simulink library "cyclopsLib"  (R2020a)
settings: Solver=VariableStepAuto  StartTime=0.0  StopTime=10.0  RelTol=1e-3
values from neighbouring files (symbols this model uses):
  agc_delay_lag = 32    [rev0BB_setup.m]
  agc_detector_coef = ones(1,agc_detector_taps)./agc_detector_taps    [rev0BB_setup.m]
  agc_sat_low = -agcSaturation    (= -12)    [rev0BB_setup.m]
  agc_sat_up = agcSaturation    (= 12)    [rev0BB_setup.m]
  agcDesired = 0    [rev0BB_setup.m]
  agcExpDomain = agcSaturation    (= 12)    [rev0BB_setup.m]
  agcExpResolution = 2^-3    (= 0.125)    [rev0BB_setup.m]
  agcPwrAvgNum = 128    [rev0BB_setup.m]
  agcSettleThresh = 0.65    [rev0BB_setup.m]
  agcStep = 2^-8    (= 0.00390625)    [rev0BB_setup.m]
  atanDomain = 5    [rev0BB_setup.m]
  atanResolution = 2^-9    (= 0.001953125)    [rev0BB_setup.m]
  bitsPerSymbolHeader = log2(radixHeader)    [rev0BB_setup.m]
  bitsPerSymbolMax = log2(radixMax)    [rev0BB_setup.m]
  cefEarlyWarning = 256    [rev0BB_setup.m]
  cefLen = length(x_CEF)    [rev0BB_setup.m]
  coarseCFOAdaptDelay = 1    [rev0BB_setup.m]
  cr_i = 0.020    (= 0.02)    [rev0BB_setup.m]
  cr_i_preamp = 2^-9    (= 0.001953125)    [rev0BB_setup.m]
  cr_int1_sat_low = -cr_integrator1_saturation    (= -0.6)    [rev0BB_setup.m]
  cr_int1_sat_up = cr_integrator1_saturation    (= 0.6)    [rev0BB_setup.m]
  cr_integrator1_decay = 1    [rev0BB_setup.m]
  cr_integrator1_saturation = 0.6    [rev0BB_setup.m]
  cr_mult_pipeline = 1    [rev0BB_setup.m]
  cr_p = 0.015    [rev0BB_setup.m]
  cr_sat2_low = -cr_saturation2    (= -0.6)    [rev0BB_setup.m]
  cr_sat2_up = cr_saturation2    (= 0.6)    [rev0BB_setup.m]
  cr_smooth_num = (1/cr_smooth_samples).*ones(1, cr_smooth_samples)    [rev0BB_setup.m]
  D_32 = [ 1,  4,  8,  2, 16]    [golay.m]    (also in rev0BB_setup.m)
  dataLenSymbols = header_len_bytes*8/bitsPerSymbolHeader + frame_len_bytes*8/bitsPerSymbol    [rev0BB_setup.m]
  delayToOutputFromDataFSM = lmsEqDepth/2-1 + regular_pipeline*9 + cr_mult_pipeline*4    (= 31)    [rev0BB_setup.m]
  enableTRFreqCorrection = true    [rev0BB_setup.m]
  expDomain = 3.3    [rev0BB_setup.m]
  expResolution = 2^-5    (= 0.03125)    [rev0BB_setup.m]
  expTol = .1    (= 0.1)    [rev0BB_setup.m]
  forceSlowRxStrobed = false    [rev0BB_setup.m]
  frac_lut_domain_cr = 64    [rev0BB_setup.m]
  frac_lut_range_max_coarse_cfo = 127    [rev0BB_setup.m]
  frac_lut_range_max_cr = 127    [rev0BB_setup.m]
  frac_lut_range_min_coarse_cfo = -frac_lut_range_max_coarse_cfo    (= -127)    [rev0BB_setup.m]
  frac_lut_range_min_cr = -frac_lut_range_max_cr    (= -127)    [rev0BB_setup.m]
  frac_lut_table_breaks_coarse_cfo = -frac_lut_domain_coarse_cfo:frac_lut_res_coarse_cfo:(frac_lut_domain_coarse_cfo-1)    [rev0BB_setup.m]
  frac_lut_table_breaks_cr = -frac_lut_domain_cr:frac_lut_res_cr:(frac_lut_domain_cr-1)    [rev0BB_setup.m]
  frac_lut_table_data_coarse_cfo = 1./frac_lut_table_breaks_coarse_cfo    [rev0BB_setup.m]
  frac_lut_table_data_cr = 1./frac_lut_table_breaks_cr    [rev0BB_setup.m]
  golay_type = 32    [rev0BB_setup.m]
  header_len_bytes = 8    [rev0BB_setup.m]
  lmsEqDepth = 38    [rev0BB_setup.m]
  lmsStep_init = 0.012    [rev0BB_setup.m]
  lmsStep_meta = (lmsStep_final - lmsStep_init)/cefLen    [rev0BB_setup.m]
  lnDomain = 16    [rev0BB_setup.m]
  lnResolution = 2^-3    (= 0.125)    [rev0BB_setup.m]
  minSTFPeaks = 3    [rev0BB_setup.m]
  mod_scheme_len_bytes = 1    [rev0BB_setup.m]
  modBPS = [1, 2, 4]    [rev0BB_setup.m]
  modKeys = [0, 1, 2]    [rev0BB_setup.m]
  mult_pipeline = 1    [rev0BB_setup.m]
  overSample = 4    [berCurve.m]    (also in rev0BB_setup.m)
  overSamplePer = 1/overSampleFreq    (= 1.25e-08)    [rev0BB_setup.m]
  qam16_demod_scale_factor = qam16_hdl_distance/qam16_power_normalized_distance    [rev0BB_setup.m]
  rcRxFilt = rcSqrtFilt    [rev0BB_setup.m]
  rcTxFilt = rcSqrtFilt    [rev0BB_setup.m]
  regular_pipeline = 1    [rev0BB_setup.m]
  rx_gain = 1    [rev0BB_setup.m]
  rx_gain_i = 1    [rev0BB_setup.m]
  rx_gain_q = 1    [rev0BB_setup.m]
  RxFeedbackPipelining = 128*3    (= 384)    [rev0BB_setup.m]
  stfLen = length(x_STF)    [rev0BB_setup.m]
  timing_differentiator_grpDelay_roundUp = ceil((timing_differentiator_len)/2)    [rev0BB_setup.m]
  timing_integrator1_decay = 0.999    [rev0BB_setup.m]
  timing_p = -1/2^2 -1/2^3    (= -0.375)    [rev0BB_setup.m]
  timing_tolerance = 4    [rev0BB_setup.m]
  timingRecoveryDoneSamplesEarly = 1    [rev0BB_setup.m]
  timingRecoveryDoneSamplesEarlyExtraDelay = -timingRecoveryDoneSamplesEarly+1    (= 0)    [rev0BB_setup.m]
  tr_int1_sat_low = -timing_integrate1_saturate    (= -0.0025)    [rev0BB_setup.m]
  tr_int1_sat_up = timing_integrate1_saturate    (= 0.0025)    [rev0BB_setup.m]
  tr_sat2_low = -timing_saturate2    (= -0.005)    [rev0BB_setup.m]
  tr_sat2_up = timing_saturate2    (= 0.005)    [rev0BB_setup.m]
  trigger = 0.40    (= 0.4)    [rev0BB_setup.m]
  trigger_tolerance = 0.35    [rev0BB_setup.m]
  W_32 = [-1,  1, -1,  1, -1]    [golay.m]    (also in rev0BB_setup.m)
  x_STFRepCount = nSpectrum_STFRepCount_short    (= 60)    [rev0BB_setup.m]
undefined symbols (not defined in the file or in its folder): agc_on, cr_integrator2_saturation, Fast_Rx_Partition, Fast_Slim_Rx_Partition, Feedback_Pipeline, freeze_en_agc, freeze_en_cr_int1, freeze_en_cr_int2, freeze_en_cr_phase, freeze_en_tr_int1, freeze_en_tr_int2, freeze_en_tr_phase, freeze_on_cef_done, freeze_on_stf_done, freeze_on_valid, i, post_cr_i_offset, post_cr_q_offset, rx_offset_correction_i, rx_offset_correction_q, Slow_Rx_Partition, timing_i, timing_i_pre_scale
libraries: simulink x62, helperLib x48, golayLib x15, commdigbbndpm3 x8, commdigbbndam3 x4, commfilt2 x3, hdlsllib x2, dspfdesign x1, simulink_need_slupdate x1, dspsigops x1, dsphdlsigops x1, $bdroot x1
(part 2 of 5)

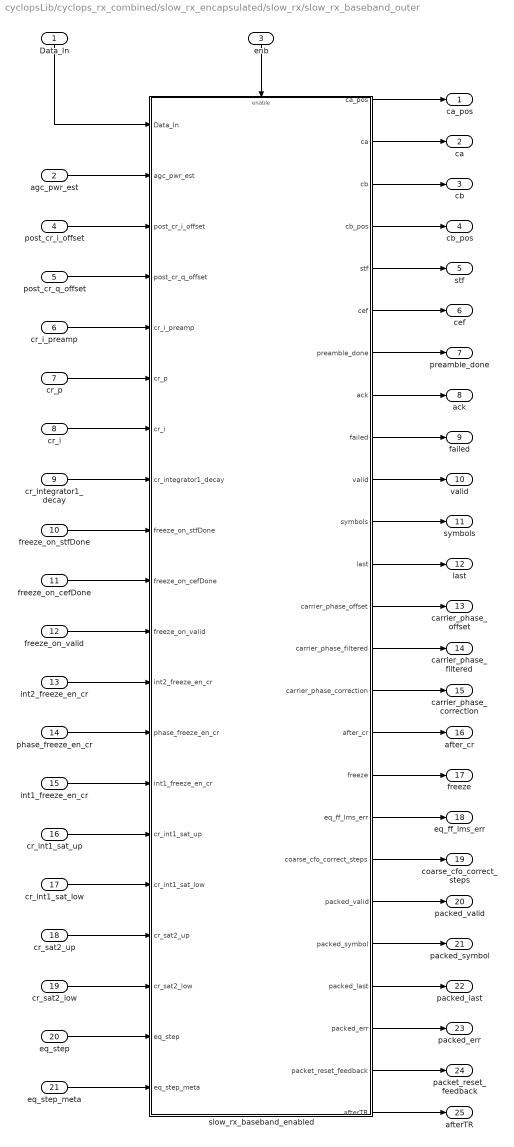
== system cyclopsLib/cyclops_rx_combined/slow_rx_encapsulated/slow_rx/slow_rx_baseband_outer ==
  Data_In : Inport
  agc_pwr_est : Inport  Port=2
  enb : Inport  Port=3
  post_cr_i_offset : Inport  Port=4
  post_cr_q_offset : Inport  Port=5
  cr_i_preamp : Inport  Port=6
  cr_p : Inport  Port=7
  cr_i : Inport  Port=8
  cr_integrator1_decay : Inport  Port=9
  freeze_on_stfDone : Inport  Port=10
  freeze_on_cefDone : Inport  Port=11
  freeze_on_valid : Inport  Port=12
  int2_freeze_en_cr : Inport  Port=13  OutDataTypeStr=boolean
  phase_freeze_en_cr : Inport  Port=14  OutDataTypeStr=boolean
  int1_freeze_en_cr : Inport  Port=15  OutDataTypeStr=boolean
  cr_int1_sat_up : Inport  Port=16
  cr_int1_sat_low : Inport  Port=17
  cr_sat2_up : Inport  Port=18
  cr_sat2_low : Inport  Port=19
  eq_step : Inport  Port=20
  eq_step_meta : Inport  Port=21
  slow_rx_baseband_enabled : Subsystem
  ca_pos : Outport  VectorParamsAs1DForOutWhenUnconnected=off
  ca : Outport  Port=2  VectorParamsAs1DForOutWhenUnconnected=off
  cb : Outport  Port=3  VectorParamsAs1DForOutWhenUnconnected=off
  cb_pos : Outport  Port=4  VectorParamsAs1DForOutWhenUnconnected=off
  stf : Outport  Port=5  VectorParamsAs1DForOutWhenUnconnected=off
  cef : Outport  Port=6  VectorParamsAs1DForOutWhenUnconnected=off
  preamble_done : Outport  Port=7  VectorParamsAs1DForOutWhenUnconnected=off
  ack : Outport  Port=8  VectorParamsAs1DForOutWhenUnconnected=off
  failed : Outport  Port=9  VectorParamsAs1DForOutWhenUnconnected=off
  valid : Outport  Port=10  VectorParamsAs1DForOutWhenUnconnected=off
  symbols : Outport  Port=11  VectorParamsAs1DForOutWhenUnconnected=off
  last : Outport  Port=12  VectorParamsAs1DForOutWhenUnconnected=off
  carrier_phase_offset : Outport  Port=13  VectorParamsAs1DForOutWhenUnconnected=off
  carrier_phase_filtered : Outport  Port=14  VectorParamsAs1DForOutWhenUnconnected=off
  carrier_phase_correction : Outport  Port=15  VectorParamsAs1DForOutWhenUnconnected=off
  after_cr : Outport  Port=16  VectorParamsAs1DForOutWhenUnconnected=off
  freeze : Outport  Port=17  VectorParamsAs1DForOutWhenUnconnected=off
  eq_ff_lms_err : Outport  Port=18  VectorParamsAs1DForOutWhenUnconnected=off
  coarse_cfo_correct_steps : Outport  Port=19  VectorParamsAs1DForOutWhenUnconnected=off
  packed_valid : Outport  Port=20  VectorParamsAs1DForOutWhenUnconnected=off
  packed_symbol : Outport  Port=21  VectorParamsAs1DForOutWhenUnconnected=off
  packed_last : Outport  Port=22  VectorParamsAs1DForOutWhenUnconnected=off
  packed_err : Outport  Port=23  VectorParamsAs1DForOutWhenUnconnected=off
  packet_reset_feedback : Outport  Port=24
  afterTR : Outport  Port=25
  wires:
  slow_rx_baseband_enabled/25(afterTR) -> afterTR/1
  slow_rx_baseband_enabled/24(packet_reset_feedback) -> packet_reset_feedback/1
  slow_rx_baseband_enabled/1(ca_pos) -> ca_pos/1
  slow_rx_baseband_enabled/2(ca) -> ca/1
  slow_rx_baseband_enabled/3(cb) -> cb/1
  slow_rx_baseband_enabled/4(cb_pos) -> cb_pos/1
  slow_rx_baseband_enabled/5(stf) -> stf/1
  slow_rx_baseband_enabled/6(cef) -> cef/1
  slow_rx_baseband_enabled/7(preamble_done) -> preamble_done/1
  slow_rx_baseband_enabled/9(failed) -> failed/1
  slow_rx_baseband_enabled/10(valid) -> valid/1
  slow_rx_baseband_enabled/11(symbols) -> symbols/1
  slow_rx_baseband_enabled/13(carrier_phase_offset) -> carrier_phase_offset/1
  slow_rx_baseband_enabled/14(carrier_phase_filtered) -> carrier_phase_filtered/1
  slow_rx_baseband_enabled/15(carrier_phase_correction) -> carrier_phase_correction/1
  Data_In/1 -> slow_rx_baseband_enabled/1(Data_In)
  enb/1 -> slow_rx_baseband_enabled/Enable
  slow_rx_baseband_enabled/16(after_cr) -> after_cr/1
  post_cr_i_offset/1 -> slow_rx_baseband_enabled/3(post_cr_i_offset)
  post_cr_q_offset/1 -> slow_rx_baseband_enabled/4(post_cr_q_offset)
  cr_i_preamp/1 -> slow_rx_baseband_enabled/5(cr_i_preamp)
  cr_p/1 -> slow_rx_baseband_enabled/6(cr_p)
  cr_i/1 -> slow_rx_baseband_enabled/7(cr_i)
  cr_integrator1_decay/1 -> slow_rx_baseband_enabled/8(cr_integrator1_decay)
  freeze_on_stfDone/1 -> slow_rx_baseband_enabled/9(freeze_on_stfDone)
  freeze_on_cefDone/1 -> slow_rx_baseband_enabled/10(freeze_on_cefDone)
  freeze_on_valid/1 -> slow_rx_baseband_enabled/11(freeze_on_valid)
  slow_rx_baseband_enabled/17(freeze) -> freeze/1
  int2_freeze_en_cr/1 -> slow_rx_baseband_enabled/12(int2_freeze_en_cr)
  cr_int1_sat_up/1 -> slow_rx_baseband_enabled/15(cr_int1_sat_up)
  cr_int1_sat_low/1 -> slow_rx_baseband_enabled/16(cr_int1_sat_low)
  cr_sat2_up/1 -> slow_rx_baseband_enabled/17(cr_sat2_up)
  cr_sat2_low/1 -> slow_rx_baseband_enabled/18(cr_sat2_low)
  phase_freeze_en_cr/1 -> slow_rx_baseband_enabled/13(phase_freeze_en_cr)
  int1_freeze_en_cr/1 -> slow_rx_baseband_enabled/14(int1_freeze_en_cr)
  slow_rx_baseband_enabled/12(last) -> last/1
  slow_rx_baseband_enabled/18(eq_ff_lms_err) -> eq_ff_lms_err/1
  agc_pwr_est/1 -> slow_rx_baseband_enabled/2(agc_pwr_est)
  eq_step/1 -> slow_rx_baseband_enabled/19(eq_step)
  eq_step_meta/1 -> slow_rx_baseband_enabled/20(eq_step_meta)
  slow_rx_baseband_enabled/19(coarse_cfo_correct_steps) -> coarse_cfo_correct_steps/1
  slow_rx_baseband_enabled/8(ack) -> ack/1
  slow_rx_baseband_enabled/20(packed_valid) -> packed_valid/1
  slow_rx_baseband_enabled/21(packed_symbol) -> packed_symbol/1
  slow_rx_baseband_enabled/22(packed_last) -> packed_last/1
  slow_rx_baseband_enabled/23(packed_err) -> packed_err/1

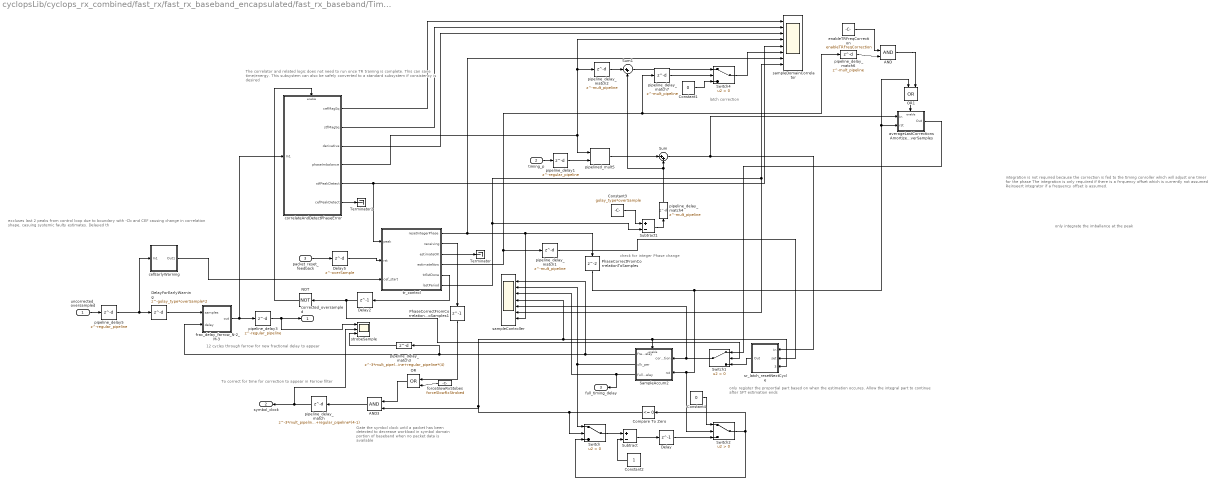
== system cyclopsLib/cyclops_rx_combined/fast_rx/fast_rx_baseband_encapsulated/fast_rx_baseband/Timing Recovery ==
  note: To correct for time for correction to appear in Farrow filter
  note: 12 cycles through farrow for new fractional delay to appear
  note: Gate the symbol clock until a packet has been
      | detected to decrease workload in symbol
      | domain portion of baseband when no packet
      | data is available
  note: only integrate the imballance at the peak
  note: integration is not required because the correction is fed to the timing conroller which will adjust one timer for the phase
      |
      | The integration is only requiired if there is a frrquency offset which is currently not assumed
      |
      | Reinseert integrator if a frequency offset is assumed.
  note: latch correction
  note: The correlator and related logic does not need to run once TR training is complete.
      | This can save time/energy.
      | This subsystem can also be safely converted to a standard subsystem if consistency is desired
  note: check for integer Phase change
  note: only register the proportial part based on when the estimation occures. Allow the integral part to continue after SFT estimation ends
  note: excluses last 2 peaks from control loop due to boundary with -Cb and CEF causing change in correlation shape, casuing
      | systemic faulty estimates.  Delayed th
  uncorrected_oversampled : Inport
  timing_p : Inport  Port=2
  packet_reset_feedback : Inport  Port=3
  AND : Logic  IconShape=distinctive  AllPortsSameDT=off  OutDataTypeStr=boolean
  AND3 : Logic  IconShape=distinctive  AllPortsSameDT=off  OutDataTypeStr=boolean
  Compare To Zero : simulink/Logic and Bit Operations/Compare To Zero  relop=<=  OutDataTypeStr=boolean
  Constant1 : Constant  Value=0  OutDataTypeStr=single
  Constant2 : Constant  OutDataTypeStr=Inherit: Inherit via back propagation  SampleTime=-1
  Constant3 : Constant  Value=golay_type*overSample  OutDataTypeStr=int32
  Constant4 : Constant  Value=0  OutDataTypeStr=single
  Delay : Delay  DelayLength=1  InitialCondition=0
  Delay2 : Delay  DelayLength=1
  Delay5 : Delay  DelayLength=overSample
  DelayForEarlyWarning : Delay  DelayLength=golay_type*overSample*2
  NOT : Logic  Operator=NOT  IconShape=distinctive  AllPortsSameDT=off  OutDataTypeStr=boolean
  OR : Logic  Operator=OR  IconShape=distinctive  AllPortsSameDT=off  OutDataTypeStr=boolean
  OR1 : Logic  Operator=OR  IconShape=distinctive  AllPortsSameDT=off  OutDataTypeStr=boolean
  PhaseCorrectFromCorrelationToSamples : Delay
  PhaseCorrectFromCorrelationToSamples1 : Delay  DelayLength=1
  SampleAccum2 : Subsystem
  Subtract : Sum  Inputs=+-  OutDataTypeStr=Inherit: Same as first input
  Subtract1 : Sum  Inputs=+-
  Sum : Sum  Inputs=|++
  Sum1 : Sum  Inputs=|++
  Switch{,1..2,4} (4 alike) : Switch  Criteria=u2 > Threshold
  Terminator : Terminator
  Terminator2 : Terminator
  averageLastCorrectionsAmortizeOverSamples : Subsystem
  cefEarlyWarning : Subsystem
  correlateAndDetectPhaseError : Subsystem
  enableTRFreqCorrection : Constant  Value=enableTRFreqCorrection  OutDataTypeStr=boolean
  forceSlowRxStobes : Constant  Value=forceSlowRxStrobed  OutDataTypeStr=boolean
  frac_delay_farrow_N-2_M-3 : Subsystem  AncestorBlock=helperLib/frac_delay_farrow_N-2_M-3  TreatAsAtomicUnit=on
  pipeline_delay1 : Delay  DelayLength=regular_pipeline
  pipeline_delay3 : Delay  DelayLength=regular_pipeline
  pipeline_delay5 : Delay  DelayLength=regular_pipeline
  pipeline_delay_match : Delay  DelayLength=3*mult_pipeline+regular_pipeline*(4-1)
  pipeline_delay_match{1..2,4,6..7} (5 alike) : Delay  DelayLength=mult_pipeline
  pipeline_delay_match3 : Delay  DelayLength=3*mult_pipeline+regular_pipeline*(4)
  pipelined_mult5 : helperLib/pipelined_mult  d=mult_pipeline
  sampleController : Scope  NumInputPorts=7
  sampleDomainCorrelator : Scope  NumInputPorts=8
  sr_latch_resetNextCycle : Subsystem
  strobeSample : Scope  NumInputPorts=3
  tr_control : Stateflow chart  TreatAsAtomicUnit=on
  corrected_oversampled : Outport  VectorParamsAs1DForOutWhenUnconnected=off
  symbol_clock : Outport  Port=2  VectorParamsAs1DForOutWhenUnconnected=off
  full_timing_delay : Outport  Port=3  VectorParamsAs1DForOutWhenUnconnected=off
  wires:
  OR1/1 -> averageLastCorrectionsAmortizeOverSamples/Enable
  enableTRFreqCorrection/1 -> AND/1
  pipeline_delay_match6/1 -> AND/2
  cefEarlyWarning/1(Out1) -> tr_control/3(cef_start)
  correlateAndDetectPhaseError/6(cefPeakDetect) -> Terminator2/1
  DelayForEarlyWarning/1 -> frac_delay_farrow_N-2_M-3/1(samples)
  frac_delay_farrow_N-2_M-3/1(out) -> pipeline_delay3/1, correlateAndDetectPhaseError/1(In1)
  pipeline_delay_match7/1 -> Switch4/2
  averageLastCorrectionsAmortizeOverSamples/1(Out) -> Switch1/1
  sr_latch_resetNextCycle/1(Out) -> Switch1/3
  AND/1 -> OR1/2
  Sum/1 -> averageLastCorrectionsAmortizeOverSamples/1(In), sr_latch_resetNextCycle/1(In)
  pipeline_delay_match4/1 -> Sum/2, Sum1/2
  Constant3/1 -> Subtract1/1
  pipeline_delay_match2/1 -> Sum1/1
  tr_control/6(lastPeriod) -> sampleDomainCorrelator/8, sampleController/6, Subtract1/2
  Subtract1/1 -> pipeline_delay_match4/1
  pipelined_mult5/1 -> Sum/1
  Switch1/1 -> SampleAccum2/1(correction), sampleController/5
  pipeline_delay_match3/1 -> strobeSample/3
  PhaseCorrectFromCorrelationToSamples1/1 -> OR/1
  PhaseCorrectFromCorrelationToSamples/1 -> Switch2/2, SampleAccum2/2(rst), averageLastCorrectionsAmortizeOverSamples/2(rst), OR1/1
  pipeline_delay3/1 -> corrected_oversampled/1, strobeSample/1
  forceSlowRxStobes/1 -> OR/2
  OR/1 -> AND3/1
  NOT/1 -> correlateAndDetectPhaseError/Enable
  Delay2/1 -> NOT/1, Switch1/2
  tr_control/5(trEstDone) -> Delay2/1
  correlateAndDetectPhaseError/3(derivative) -> sampleDomainCorrelator/3
  correlateAndDetectPhaseError/2(stfMagSq) -> sampleDomainCorrelator/2
  correlateAndDetectPhaseError/1(cefMagSq) -> sampleDomainCorrelator/1
  correlateAndDetectPhaseError/5(stfPeakDetect) -> tr_control/1(peak), sampleDomainCorrelator/5
  correlateAndDetectPhaseError/4(phaseImbalance) -> pipelined_mult5/1, sampleDomainCorrelator/4, pipeline_delay_match2/1
  tr_control/3(estimateOK) -> Terminator/1
  Delay5/1 -> tr_control/2(rst)
  pipeline_delay_match/1 -> strobeSample/2, symbol_clock/1
  AND3/1 -> pipeline_delay_match/1
  Sum1/1 -> Switch4/1
  Switch4/1 -> sampleDomainCorrelator/6
  Constant4/1 -> Switch2/1
  Delay/1 -> Switch2/3
  pipeline_delay1/1 -> pipelined_mult5/2
  Constant1/1 -> Switch4/3
  pipeline_delay_match1/1 -> sr_latch_resetNextCycle/2(set)
  timing_p/1 -> pipeline_delay1/1
  tr_control/1(resetIntegerPhase) -> PhaseCorrectFromCorrelationToSamples/1, sampleController/7, sampleDomainCorrelator/7
  tr_control/2(receiving) -> PhaseCorrectFromCorrelationToSamples1/1
  tr_control/4(estimateNow) -> pipeline_delay_match1/1, pipeline_delay_match6/1, pipeline_delay_match7/1
  packet_reset_feedback/1 -> Delay5/1
  Switch2/1 -> Compare To Zero/1, Switch/3
  Switch/1 -> Subtract/1
  Constant2/1 -> Subtract/2
  SampleAccum2/2(clk_per) -> sampleController/2, Switch/1
  Subtract/1 -> Delay/1
  uncorrected_oversampled/1 -> pipeline_delay5/1
  SampleAccum2/3(fullDelay) -> sampleController/3, full_timing_delay/1
  Compare To Zero/1 -> Switch/2, AND3/2, sampleController/4, SampleAccum2/Enable, sr_latch_resetNextCycle/3(rst_next)
  SampleAccum2/1(fracDelay) -> sampleController/1, frac_delay_farrow_N-2_M-3/2(delay), pipeline_delay_match3/1
  pipeline_delay5/1 -> DelayForEarlyWarning/1, cefEarlyWarning/1(In1)

== system cyclopsLib/cyclops_rx_combined/fast_rx/fast_rx_baseband_slim_encapsulated/slim_fast_rx/AGC ==
  note: Intentionally let width grow due to distinct chance of overflow
  In : Inport
  Desired : Inport  Port=2
  Step : Inport  Port=3
  freeze : Inport  Port=4  OutDataTypeStr=boolean
  agc_sat_up : Inport  Port=5
  agc_sat_low : Inport  Port=6
  Compare To Constant : simulink/Logic and Bit Operations/Compare To Constant  relop=<  const=lnResolution  OutDataTypeStr=boolean
  Constant : Constant  Value=lnResolution  OutDataTypeStr=Inherit: Inherit via back propagation
  Data Type Duplicate1 : DataTypeDuplicate
  Data Type Conversion1 : DataTypeConversion  OutDataTypeStr=single
  Delay : Delay  DelayLength=1  InitialCondition=0
  Discrete FIR Filter : DiscreteFir  FilterStructure=Direct form transposed  Coefficients=agc_detector_coef  InputProcessing=Columns as channels (frame based)  OutDataTypeStr=Inherit: Same as input
  Exp : Math  SignedPower=on  SaturateOnIntegerOverflow=on
  Log : Math  Operator=log  SignedPower=on  SaturateOnIntegerOverflow=on
  Saturation Dynamic : simulink/Discontinuities/Saturation Dynamic  OutMin=[]  OutMax=[]  OutDataTypeStr=Inherit: Same as second input  OutDataType=fixdt(1, 16)  OutScaling=2^-10  DoSatur=off
  Sum : Sum  Inputs=-+  OutDataTypeStr=Inherit: Same as first input
  Sum1 : Sum  Inputs=|++  OutDataTypeStr=Inherit: Same as first input
  Switch : Switch  Criteria=u2 > Threshold
  Switch1 : Switch  Criteria=u2 > Threshold
  complex_magnitude_sq_cfg : helperLib/complex_magnitude_sq_cfg  mult=0  pipe=0
  exp : Subsystem  Commented=on
  ln1 : Subsystem  Commented=on
  pipelined_mult2 : helperLib/pipelined_mult  d=0
  Correction : Outport  VectorParamsAs1DForOutWhenUnconnected=off
  LnPwr : Outport  Port=2  VectorParamsAs1DForOutWhenUnconnected=off
  AfterFilter : Outport  Port=3  VectorParamsAs1DForOutWhenUnconnected=off
  wires:
  In/1 -> Data Type Conversion1/1
  Sum/1 -> pipelined_mult2/2
  Step/1 -> pipelined_mult2/1
  Sum1/1 -> Switch1/3
  Exp/1 -> Data Type Duplicate1/1, Correction/1
  Log/1 -> LnPwr/1, Sum/1
  Desired/1 -> Sum/2
  Discrete FIR Filter/1 -> AfterFilter/1, Switch/3, Compare To Constant/1, Data Type Duplicate1/2
  pipelined_mult2/1 -> Sum1/1
  Delay/1 -> Switch1/1, Saturation Dynamic/2
  complex_magnitude_sq_cfg/1 -> Discrete FIR Filter/1
  Data Type Conversion1/1 -> complex_magnitude_sq_cfg/1
  freeze/1 -> Switch1/2
  agc_sat_low/1 -> Saturation Dynamic/3
  agc_sat_up/1 -> Saturation Dynamic/1
  Saturation Dynamic/1 -> Sum1/2, Exp/1
  Switch1/1 -> Delay/1
  Switch/1 -> Log/1
  Compare To Constant/1 -> Switch/2
  Constant/1 -> Switch/1

== system cyclopsLib/cyclops_rx_combined/fast_rx/fast_rx_baseband_slim_encapsulated/slim_fast_rx/RxRaisedCosine2 ==
  note: Note: the tool should optomize a single FIR filter to this config due to 0 propogation. However, will make explicit for now
  note: (a+bj)(c+dj) = ac+adj+bcj-bd
      | If d = 0 | = ac + bcj
  note: Raised Cosine Filter Can be Split because it is Real (use 2 multiplies instead of 4 per tap)
  In2 : Inport
  Complex to Real-Imag : ComplexToRealImag
  Discrete FIR Filter : DiscreteFir  FilterStructure=Direct form transposed  Coefficients=rcRxFilt  AccumDataTypeStr=Inherit: Same as product output
  Discrete FIR Filter1 : DiscreteFir  FilterStructure=Direct form transposed  Coefficients=rcRxFilt  AccumDataTypeStr=Inherit: Same as product output
  Raised Cosine Receive Filter : commfilt2/Raised Cosine Receive Filter  Commented=on  filtType=Square root  R=.1  filtSpan=16  N=4  downFactor=1  downOffset=0  filterGain=1  InputProcessing=Columns as channels (frame based)  RateOptions=Enforce single-rate processing  framing=Mute  checkCoeff=on  variableName=rcRxFilt  currentFiltSpan=16  D=(16)/2  inputOffset=0  sampMode=Mute  saveAsFlag=0  rateMode=Downsampling  checkGain=Normalized  launchFVT=on  roundingMode=Floor  overflowMode=off  coeffDataTypeStr=Inherit: Same word length as input  coeffMin=[]  coeffMax=[]  coeffLastDataTypeStr=Inherit: Same word length as input  accumDataTypeStr=Inherit: Same as product output  accumLastDataTypeStr=Inherit: Same as product output  outputDataTypeStr=Inherit: Same as accumulator  outputMin=[]  outputMax=[]  outputLastDataTypeStr=Inherit: Same as accumulator
  Real-Imag to Complex : RealImagToComplex
  Out2 : Outport  VectorParamsAs1DForOutWhenUnconnected=off
  wires:
  In2/1 -> Complex to Real-Imag/1
  Complex to Real-Imag/1 -> Discrete FIR Filter/1
  Complex to Real-Imag/2 -> Discrete FIR Filter1/1
  Discrete FIR Filter/1 -> Real-Imag to Complex/1
  Discrete FIR Filter1/1 -> Real-Imag to Complex/2
  Real-Imag to Complex/1 -> Out2/1

== system cyclopsLib/cyclops_rx_combined/fast_rx/fast_rx_baseband_slim_encapsulated/slim_fast_rx/average_filter ==
  note: Clever Arch of an Averaging Filter I saw in A Split MAC Approach for SDR Platforms by Paolo Di Francesco, S´eamas McGettrick, Uchenna K. Anyanwu, James C. O’Sullivan,
      | Allen B. MacKenzie, and Luiz A. DaSilva.  This requires a shift register, 1 mult, and 2 adds (3 if you count the negation).  Downside is unpipelined loopback (standard IIR problem)
  In1 : Inport
  Data Type Conversion : DataTypeConversion
  Delay : Delay  DelayLength=samples  InitialCondition=0
  Delay1 : Delay  DelayLength=1  InitialCondition=0
  Gain : Gain  Gain=gain  OutDataTypeStr=Inherit: Same as input
  Sum : Sum  Inputs=|++  OutDataTypeStr=Inherit: Same as first input
  Sum1 : Sum  Inputs=|+-  OutDataTypeStr=Inherit: Same as first input
  pipeline_delay : Delay  DelayLength=pipe
  Out1 : Outport  VectorParamsAs1DForOutWhenUnconnected=off
  wires:
  Data Type Conversion/1 -> Sum/1
  pipeline_delay/1 -> Data Type Conversion/1, Delay/1
  Gain/1 -> pipeline_delay/1
  Delay1/1 -> Sum/2
  Sum1/1 -> Delay1/1, Out1/1
  Delay/1 -> Sum1/2
  In1/1 -> Gain/1
  Sum/1 -> Sum1/1

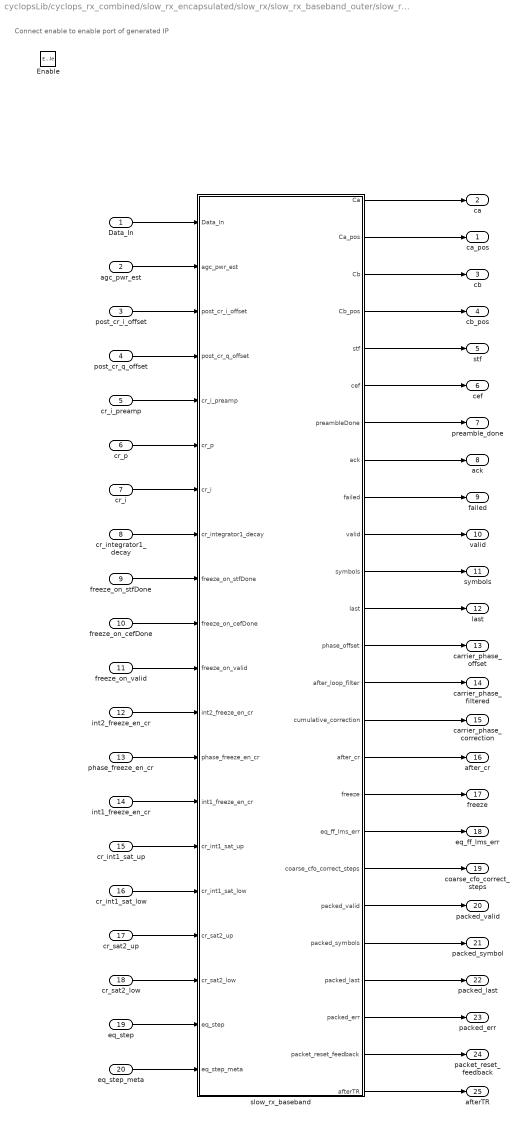
== system cyclopsLib/cyclops_rx_combined/slow_rx_encapsulated/slow_rx/slow_rx_baseband_outer/slow_rx_baseband_enabled ==
  note: Connect enable to enable port of generated IP
  Data_In : Inport
  agc_pwr_est : Inport  Port=2
  post_cr_i_offset : Inport  Port=3
  post_cr_q_offset : Inport  Port=4
  cr_i_preamp : Inport  Port=5
  cr_p : Inport  Port=6
  cr_i : Inport  Port=7
  cr_integrator1_decay : Inport  Port=8
  freeze_on_stfDone : Inport  Port=9
  freeze_on_cefDone : Inport  Port=10
  freeze_on_valid : Inport  Port=11
  int2_freeze_en_cr : Inport  Port=12  OutDataTypeStr=boolean
  phase_freeze_en_cr : Inport  Port=13  OutDataTypeStr=boolean
  int1_freeze_en_cr : Inport  Port=14  OutDataTypeStr=boolean
  cr_int1_sat_up : Inport  Port=15
  cr_int1_sat_low : Inport  Port=16
  cr_sat2_up : Inport  Port=17
  cr_sat2_low : Inport  Port=18
  eq_step : Inport  Port=19
  eq_step_meta : Inport  Port=20
  Enable : EnablePort
  slow_rx_baseband : Subsystem
  ca_pos : Outport  InitialOutput=0  VectorParamsAs1DForOutWhenUnconnected=off
  ca : Outport  Port=2  InitialOutput=0  VectorParamsAs1DForOutWhenUnconnected=off
  cb : Outport  Port=3  InitialOutput=0  VectorParamsAs1DForOutWhenUnconnected=off
  cb_pos : Outport  Port=4  InitialOutput=0  VectorParamsAs1DForOutWhenUnconnected=off
  stf : Outport  Port=5  InitialOutput=0  VectorParamsAs1DForOutWhenUnconnected=off
  cef : Outport  Port=6  InitialOutput=0  VectorParamsAs1DForOutWhenUnconnected=off
  preamble_done : Outport  Port=7  InitialOutput=0  VectorParamsAs1DForOutWhenUnconnected=off
  ack : Outport  Port=8  InitialOutput=0  VectorParamsAs1DForOutWhenUnconnected=off
  failed : Outport  Port=9  InitialOutput=0  VectorParamsAs1DForOutWhenUnconnected=off
  valid : Outport  Port=10  InitialOutput=0  VectorParamsAs1DForOutWhenUnconnected=off
  symbols : Outport  Port=11  InitialOutput=0  VectorParamsAs1DForOutWhenUnconnected=off
  last : Outport  Port=12  InitialOutput=[0]  VectorParamsAs1DForOutWhenUnconnected=off
  carrier_phase_offset : Outport  Port=13  InitialOutput=0  VectorParamsAs1DForOutWhenUnconnected=off
  carrier_phase_filtered : Outport  Port=14  InitialOutput=0  VectorParamsAs1DForOutWhenUnconnected=off
  carrier_phase_correction : Outport  Port=15  InitialOutput=0  VectorParamsAs1DForOutWhenUnconnected=off
  after_cr : Outport  Port=16  InitialOutput=0  VectorParamsAs1DForOutWhenUnconnected=off
  freeze : Outport  Port=17  InitialOutput=[0]  VectorParamsAs1DForOutWhenUnconnected=off
  eq_ff_lms_err : Outport  Port=18  InitialOutput=0  VectorParamsAs1DForOutWhenUnconnected=off
  coarse_cfo_correct_steps : Outport  Port=19  InitialOutput=0  VectorParamsAs1DForOutWhenUnconnected=off
  packed_valid : Outport  Port=20  InitialOutput=0  VectorParamsAs1DForOutWhenUnconnected=off
  packed_symbol : Outport  Port=21  InitialOutput=0  VectorParamsAs1DForOutWhenUnconnected=off
  packed_last : Outport  Port=22  InitialOutput=0  VectorParamsAs1DForOutWhenUnconnected=off
  packed_err : Outport  Port=23  InitialOutput=0  VectorParamsAs1DForOutWhenUnconnected=off
  packet_reset_feedback : Outport  Port=24
  afterTR : Outport  Port=25
  wires:
  slow_rx_baseband/25(afterTR) -> afterTR/1
  slow_rx_baseband/24(packet_reset_feedback) -> packet_reset_feedback/1
  slow_rx_baseband/1(Ca) -> ca/1
  slow_rx_baseband/2(Ca_pos) -> ca_pos/1
  slow_rx_baseband/3(Cb) -> cb/1
  slow_rx_baseband/4(Cb_pos) -> cb_pos/1
  slow_rx_baseband/5(stf) -> stf/1
  slow_rx_baseband/6(cef) -> cef/1
  slow_rx_baseband/7(preambleDone) -> preamble_done/1
  slow_rx_baseband/9(failed) -> failed/1
  slow_rx_baseband/10(valid) -> valid/1
  slow_rx_baseband/11(symbols) -> symbols/1
  slow_rx_baseband/13(phase_offset) -> carrier_phase_offset/1
  slow_rx_baseband/14(after_loop_filter) -> carrier_phase_filtered/1
  slow_rx_baseband/15(cumulative_correction) -> carrier_phase_correction/1
  Data_In/1 -> slow_rx_baseband/1(Data_In)
  slow_rx_baseband/16(after_cr) -> after_cr/1
  post_cr_i_offset/1 -> slow_rx_baseband/3(post_cr_i_offset)
  post_cr_q_offset/1 -> slow_rx_baseband/4(post_cr_q_offset)
  cr_i_preamp/1 -> slow_rx_baseband/5(cr_i_preamp)
  cr_p/1 -> slow_rx_baseband/6(cr_p)
  cr_i/1 -> slow_rx_baseband/7(cr_i)
  cr_integrator1_decay/1 -> slow_rx_baseband/8(cr_integrator1_decay)
  freeze_on_stfDone/1 -> slow_rx_baseband/9(freeze_on_stfDone)
  freeze_on_cefDone/1 -> slow_rx_baseband/10(freeze_on_cefDone)
  freeze_on_valid/1 -> slow_rx_baseband/11(freeze_on_valid)
  slow_rx_baseband/17(freeze) -> freeze/1
  int2_freeze_en_cr/1 -> slow_rx_baseband/12(int2_freeze_en_cr)
  cr_int1_sat_up/1 -> slow_rx_baseband/15(cr_int1_sat_up)
  cr_int1_sat_low/1 -> slow_rx_baseband/16(cr_int1_sat_low)
  cr_sat2_up/1 -> slow_rx_baseband/17(cr_sat2_up)
  cr_sat2_low/1 -> slow_rx_baseband/18(cr_sat2_low)
  phase_freeze_en_cr/1 -> slow_rx_baseband/13(phase_freeze_en_cr)
  int1_freeze_en_cr/1 -> slow_rx_baseband/14(int1_freeze_en_cr)
  slow_rx_baseband/12(last) -> last/1
  slow_rx_baseband/18(eq_ff_lms_err) -> eq_ff_lms_err/1
  agc_pwr_est/1 -> slow_rx_baseband/2(agc_pwr_est)
  eq_step/1 -> slow_rx_baseband/19(eq_step)
  eq_step_meta/1 -> slow_rx_baseband/20(eq_step_meta)
  slow_rx_baseband/19(coarse_cfo_correct_steps) -> coarse_cfo_correct_steps/1
  slow_rx_baseband/8(ack) -> ack/1
  slow_rx_baseband/20(packed_valid) -> packed_valid/1
  slow_rx_baseband/21(packed_symbols) -> packed_symbol/1
  slow_rx_baseband/22(packed_last) -> packed_last/1
  slow_rx_baseband/23(packed_err) -> packed_err/1

== system cyclopsLib/cyclops_rx_combined/fast_rx/fast_rx_baseband_encapsulated/fast_rx_baseband/Timing Recovery/SampleAccum2 ==
  note: Based on Digital Communication Recievers by Meyr pg 530 but modified
      |
      | The error here is in "samples". The correction input is in fact -error and
      | dictates how the clock should be changed.
      |
      | The clk_per is not simply the integer portion of the delay, which is
      | somewhat counterintuitive. This is because the clk_per line is controling
      | the delay for the rx clk (in terms of samples). Here is some intuition:
      | Say that the desired phase is exactly on a sample (fractional delay = 0).
      | One can get the same phase by setting the fractional phase to 1 but the
      | clock must add 1 sample to catch up with the additional delay added.
      |
      | The same logic holds true in the reverse case. Delay can be changed
      | from 1 to 0 but the clock must skip a sample to catch up.
      |
      | Diagrams showing the clock logic as well as the logic when a phase correction
      | is non-zeros are presented to the left of this text.
  note: Division Represented as Shift
  note: Initial Fractional delay was changed to 0.5 because, unless the
      | peak changes position, the correction is either fractional increase
      | or fractional decrease.
  correction : Inport
  rst : Inport  Port=2  OutDataTypeStr=boolean
  Enable : EnablePort
  Add1 : Sum  OutDataTypeStr=Inherit: Same as first input
  Add2 : Sum  OutDataTypeStr=Inherit: Same as first input
  Add4 : Sum  OutDataTypeStr=Inherit: Same as first input
  Constant : Constant  Value=0.5  OutDataTypeStr=Inherit: Inherit via back propagation
  Constant3 : Constant  Value=4  OutDataTypeStr=Inherit: Inherit via back propagation  SampleTime=-1
  Constant4 : Constant  Value=4  OutDataTypeStr=Inherit: Inherit via back propagation  SampleTime=-1
  Data Type Conversion1 : DataTypeConversion  OutDataTypeStr=int8
  Data Type Conversion2 : DataTypeConversion
  Data Type Conversion3 : DataTypeConversion
  Delay2 : Delay  DelayLength=1  InitialCondition=0.5
  Gain : Gain  Gain=-1  OutDataTypeStr=Inherit: Same as input
  Sub2 : Sum  Inputs=+-  OutDataTypeStr=Inherit: Same as first input
  Sub3 : Sum  Inputs=+-  OutDataTypeStr=Inherit: Same as first input
  Switch : Switch  Criteria=u2 > Threshold  OutDataTypeStr=Inherit: Inherit via back propagation
  fracDelay : Outport  InitialOutput=[0]  VectorParamsAs1DForOutWhenUnconnected=off
  clk_per : Outport  Port=2  InitialOutput=[0]  VectorParamsAs1DForOutWhenUnconnected=off
  fullDelay : Outport  Port=3  InitialOutput=[0]  VectorParamsAs1DForOutWhenUnconnected=off
  wires:
  Constant/1 -> Switch/1
  Delay2/1 -> Switch/3
  Sub2/1 -> fracDelay/1, Delay2/1
  rst/1 -> Switch/2
  Sub3/1 -> Gain/1
  Constant3/1 -> Add1/2
  Data Type Conversion1/1 -> Sub3/1, Data Type Conversion2/1
  Switch/1 -> Add2/2
  Add2/1 -> fullDelay/1, Data Type Conversion3/1, Data Type Conversion1/1
  Add4/1 -> clk_per/1
  Constant4/1 -> Add4/2, Sub3/2
  correction/1 -> Add1/1
  Gain/1 -> Add4/1
  Add1/1 -> Add2/1
  Data Type Conversion2/1 -> Sub2/2
  Data Type Conversion3/1 -> Sub2/1

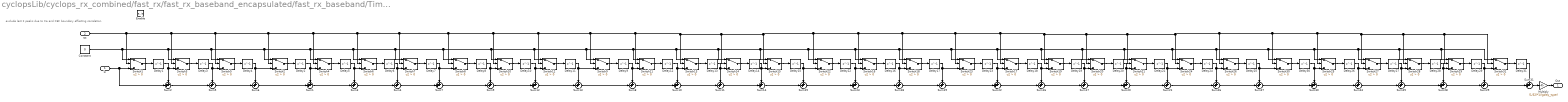
== system cyclopsLib/cyclops_rx_combined/fast_rx/fast_rx_baseband_encapsulated/fast_rx_baseband/Timing Recovery/averageLastCorrectionsAmortizeOverSamples ==
  note: exclude last 2 peaks due to Ca and CEF boundary effecting correlation
  In : Inport
  rst : Inport  Port=2
  Enable : EnablePort
  Constant : Constant  Value=0  OutDataTypeStr=single
  Delay{1..31} (31 alike) : Delay  DelayLength=1
  Multiply : Gain  Gain=(1/32)*1/(golay_type)
  Sum{1..31} (31 alike) : Sum  Inputs=++|
  Switch{1..31} (31 alike) : Switch  Criteria=u2 > Threshold
  Out : Outport  InitialOutput=[0]
  wires:
  Sum31/1 -> Multiply/1
  Delay29/1 -> Sum29/1, Switch31/3
  Switch31/1 -> Delay31/1
  Delay31/1 -> Sum31/1
  Sum29/1 -> Sum31/2
  Switch25/1 -> Delay26/1
  Delay26/1 -> Sum24/1, Switch27/3
  Delay21/1 -> Sum21/1, Switch24/3
  Switch27/1 -> Delay27/1
  Sum30/1 -> Sum24/2
  Switch26/1 -> Delay25/1
  Delay25/1 -> Sum27/1, Switch30/3
  Sum25/1 -> Sum28/2
  Delay27/1 -> Sum25/1, Switch28/3
  Delay28/1 -> Sum28/1, Switch29/3
  rst/1 -> Switch1/2, Switch3/2, Switch5/2, Switch2/2, Switch4/2, Switch12/2, Switch9/2, Switch11/2, Switch13/2, Switch14/2, Switch15/2, Switch18/2, Switch23/2, Switch17/2, Switch19/2, Switch20/2, Switch21/2, Switch24/2, Switch26/2, Switch30/2, Switch25/2, Switch27/2, Switch28/2, Switch31/2, Switch29/2, Switch16/2, Switch22/2, Switch10/2, Switch8/2, Switch7/2, Switch6/2
  Sum28/1 -> Sum29/2
  Sum27/1 -> Sum30/2
  Switch30/1 -> Delay30/1
  Delay24/1 -> Sum26/1, Switch26/3
  Switch28/1 -> Delay28/1
  Switch24/1 -> Delay24/1
  Sum24/1 -> Sum25/2
  Constant/1 -> Switch1/1, Switch3/1, Switch5/1, Switch2/1, Switch4/1, Switch7/1, Switch10/1, Switch12/1, Switch9/1, Switch11/1, Switch15/1, Switch16/1, Switch18/1, Switch23/1, Switch17/1, Switch26/1, Switch30/1, Switch25/1, Switch29/1, Switch31/1, Switch28/1, Switch27/1, Switch24/1, Switch21/1, Switch20/1, Switch19/1, Switch22/1, Switch14/1, Switch13/1, Switch8/1, Switch6/1
  Switch29/1 -> Delay29/1
  Delay30/1 -> Switch25/3, Sum30/1
  Sum21/1 -> Sum26/2
  Sum26/1 -> Sum27/2
  Sum15/1 -> Sum23/2
  Delay19/1 -> Sum17/1, Switch20/3
  Sum22/1 -> Sum16/2
  Switch17/1 -> Delay18/1
  Sum16/1 -> Sum17/2
  Delay18/1 -> Sum16/1, Switch19/3
  Switch18/1 -> Delay17/1
  Delay22/1 -> Switch16/3, Sum23/1
  Switch20/1 -> Delay20/1
  Delay20/1 -> Sum20/1, Switch21/3
  Switch19/1 -> Delay19/1
  Delay17/1 -> Sum19/1, Switch23/3
  Sum18/1 -> Sum19/2
  Sum20/1 -> Sum21/2
  Switch23/1 -> Delay23/1
  Switch16/1 -> Delay16/1
  Switch22/1 -> Delay22/1
  Delay16/1 -> Sum18/1, Switch18/3
  Delay23/1 -> Switch17/3, Sum22/1
  Sum17/1 -> Sum20/2
  Switch21/1 -> Delay21/1
  Sum19/1 -> Sum22/2
  Sum23/1 -> Sum18/2
  Sum14/1 -> Sum15/2
  Switch15/1 -> Delay15/1
  Delay15/1 -> Sum15/1, Switch22/3
  Sum7/1 -> Sum9/2
  Delay13/1 -> Sum11/1, Switch14/3
  Delay12/1 -> Sum10/1, Switch13/3
  Switch14/1 -> Delay14/1
  Delay8/1 -> Switch10/3, Sum9/1
  Sum11/1 -> Sum14/2
  Sum8/1 -> Sum10/2
  Switch11/1 -> Delay12/1
  Switch12/1 -> Delay11/1
  Switch13/1 -> Delay13/1
  Sum10/1 -> Sum11/2
  Delay11/1 -> Sum13/1, Switch9/3
  Delay14/1 -> Sum14/1, Switch15/3
  Sum12/1 -> Sum13/2
  Delay10/1 -> Sum12/1, Switch12/3
  Switch10/1 -> Delay10/1
  Switch9/1 -> Delay9/1
  Delay9/1 -> Switch11/3, Sum8/1
  Sum13/1 -> Sum8/2
  Sum9/1 -> Sum12/2
  Switch8/1 -> Delay8/1
  Delay7/1 -> Sum7/1, Switch8/3
  Switch7/1 -> Delay7/1
  Sum4/1 -> Sum7/2
  Sum6/1 -> Sum1/2
  Delay4/1 -> Sum6/1, Switch2/3
  Switch6/1 -> Delay6/1
  Delay5/1 -> Sum3/1, Switch6/3
  Delay6/1 -> Sum4/1, Switch7/3
  Sum3/1 -> Sum4/2
  Delay2/1 -> Switch4/3, Sum1/1
  Switch4/1 -> Delay5/1
  Sum1/1 -> Sum3/2
  Switch2/1 -> Delay2/1
  In/1 -> Sum2/2, Switch1/3
  Multiply/1 -> Out/1
  Delay3/1 -> Sum5/1, Switch5/3
  Switch5/1 -> Delay4/1
  Delay1/1 -> Switch3/3, Sum2/1
  Sum2/1 -> Sum5/2
  Switch3/1 -> Delay3/1
  Sum5/1 -> Sum6/2
  Switch1/1 -> Delay1/1

== system cyclopsLib/cyclops_rx_combined/fast_rx/fast_rx_baseband_encapsulated/fast_rx_baseband/Timing Recovery/cefEarlyWarning ==
  In1 : Inport
  AND5 : Logic  IconShape=distinctive  AllPortsSameDT=off  OutDataTypeStr=boolean
  Compare To Constant5 : simulink/Logic and Bit Operations/Compare To Constant  relop=<  const=1+trigger  OutDataTypeStr=boolean
  Compare To Constant6 : simulink/Logic and Bit Operations/Compare To Constant  relop=>=  const=trigger  OutDataTypeStr=boolean
  Complex to Real-Imag2 : ComplexToRealImag
  Constant5 : Constant  Value=1/golay_type  OutDataTypeStr=Inherit: Inherit via back propagation  SampleTime=-1
  Delay3 : Delay  DelayLength=timing_differentiator_grpDelay_roundUp
  Golay Correlator 32 : Subsystem  TreatAsAtomicUnit=on
  Real-Imag to Complex1 : RealImagToComplex
  Terminator1 : Terminator
  complex_magnitude_sq_cfg : helperLib/complex_magnitude_sq_cfg  mult=mult_pipeline  pipe=regular_pipeline
  pipelined_mult1 : helperLib/pipelined_mult  d=mult_pipeline
  pipelined_mult2 : helperLib/pipelined_mult  d=mult_pipeline
  Out1 : Outport
  wires:
  Compare To Constant6/1 -> AND5/1
  Golay Correlator 32/1(Ca) -> Complex to Real-Imag2/1
  pipelined_mult2/1 -> Real-Imag to Complex1/2
  Constant5/1 -> pipelined_mult1/2, pipelined_mult2/2
  AND5/1 -> Out1/1
  Delay3/1 -> Compare To Constant6/1, Compare To Constant5/1
  pipelined_mult1/1 -> Real-Imag to Complex1/1
  Real-Imag to Complex1/1 -> complex_magnitude_sq_cfg/1
  Complex to Real-Imag2/2 -> pipelined_mult2/1
  Compare To Constant5/1 -> AND5/2
  complex_magnitude_sq_cfg/1 -> Delay3/1
  Complex to Real-Imag2/1 -> pipelined_mult1/1
  Golay Correlator 32/2(Cb) -> Terminator1/1
  In1/1 -> Golay Correlator 32/1(In)

== system cyclopsLib/cyclops_rx_combined/fast_rx/fast_rx_baseband_encapsulated/fast_rx_baseband/Timing Recovery/correlateAndDetectPhaseError ==
  note: Detect Zero Crossing of Phase
  note: Detect the peak (within thresholdRange) and slope changes from + to -)
  note: detect the imballance
  In1 : Inport
  Enable : EnablePort
  AND{,1,4..5} (4 alike) : Logic  IconShape=distinctive  AllPortsSameDT=off  OutDataTypeStr=boolean
  Add : Sum
  Compare To Constant1 : simulink/Logic and Bit Operations/Compare To Constant  relop=<  const=1+trigger  OutDataTypeStr=boolean
  Compare To Constant2 : simulink/Logic and Bit Operations/Compare To Constant  relop=>=  const=0  OutDataTypeStr=boolean
  Compare To Constant3 : simulink/Logic and Bit Operations/Compare To Constant  relop=<  const=0  OutDataTypeStr=boolean
  Compare To Constant4 : simulink/Logic and Bit Operations/Compare To Constant  relop=>=  const=trigger  OutDataTypeStr=boolean
  Compare To Constant5 : simulink/Logic and Bit Operations/Compare To Constant  relop=<  const=1+trigger  OutDataTypeStr=boolean
  Compare To Constant6 : simulink/Logic and Bit Operations/Compare To Constant  relop=>=  const=trigger  OutDataTypeStr=boolean
  Complex to Real-Imag2 : ComplexToRealImag
  Complex to Real-Imag3 : ComplexToRealImag
  Constant3 : Constant  Value=1/golay_type  OutDataTypeStr=Inherit: Inherit via back propagation  SampleTime=-1
  Delay2 : Delay  DelayLength=timing_differentiator_grpDelay_roundUp
  Delay3 : Delay  DelayLength=timing_differentiator_grpDelay_roundUp
  Delay4 : Delay  DelayLength=1
  Differentiator Filter : dspfdesign/Differentiator Filter  DesignForMinimumOrder=off  FilterOrder=timing_differentiator_len  PassbandRipple=0.1  ScaleCoefficients=off  SimulateUsing=Interpreted execution  roundingMode=Floor  coeffsDataTypeStr=fixdt(1,16)
      settings: SourceProductBaseCode=DS
  Golay Correlator 32 : Subsystem  TreatAsAtomicUnit=on
  Real-Imag to Complex1 : RealImagToComplex
  Real-Imag to Complex2 : RealImagToComplex
  complex_magnitude_sq_cfg : helperLib/complex_magnitude_sq_cfg  mult=mult_pipeline  pipe=regular_pipeline
  complex_magnitude_sq_cfg1 : helperLib/complex_magnitude_sq_cfg  mult=mult_pipeline  pipe=regular_pipeline
  pipelined_mult{1..4} (4 alike) : helperLib/pipelined_mult  d=mult_pipeline
  cefMagSq : Outport
  stfMagSq : Outport  Port=2
  derivative : Outport  Port=3
  phaseImbalance : Outport  Port=4
  stfPeakDetect : Outport  Port=5
  cefPeakDetect : Outport  Port=6
  wires:
  Compare To Constant5/1 -> AND5/2
  Complex to Real-Imag3/1 -> pipelined_mult3/1
  Compare To Constant6/1 -> AND5/1
  AND5/1 -> cefPeakDetect/1
  Delay2/1 -> Compare To Constant4/1, Compare To Constant1/1, stfMagSq/1
  pipelined_mult4/1 -> Real-Imag to Complex2/2
  Delay3/1 -> Compare To Constant5/1, Compare To Constant6/1, cefMagSq/1
  pipelined_mult1/1 -> Real-Imag to Complex1/1
  Constant3/1 -> pipelined_mult3/2, pipelined_mult4/2, pipelined_mult1/2, pipelined_mult2/2
  pipelined_mult3/1 -> Real-Imag to Complex2/1
  Golay Correlator 32/1(Ca) -> Complex to Real-Imag2/1
  Compare To Constant1/1 -> AND4/2
  Compare To Constant4/1 -> AND4/1
  complex_magnitude_sq_cfg1/1 -> Delay2/1, Differentiator Filter/1
  AND1/1 -> stfPeakDetect/1
  pipelined_mult2/1 -> Real-Imag to Complex1/2
  Real-Imag to Complex1/1 -> complex_magnitude_sq_cfg/1
  Differentiator Filter/1 -> Delay4/1, Compare To Constant3/1, Add/1, derivative/1
  Complex to Real-Imag3/2 -> pipelined_mult4/1
  Golay Correlator 32/2(Cb) -> Complex to Real-Imag3/1
  Complex to Real-Imag2/2 -> pipelined_mult2/1
  Complex to Real-Imag2/1 -> pipelined_mult1/1
  complex_magnitude_sq_cfg/1 -> Delay3/1
  Real-Imag to Complex2/1 -> complex_magnitude_sq_cfg1/1
  Compare To Constant2/1 -> AND/2
  Delay4/1 -> Add/2, Compare To Constant2/1
  Compare To Constant3/1 -> AND/1
  Add/1 -> phaseImbalance/1
  AND4/1 -> AND1/2
  AND/1 -> AND1/1
  In1/1 -> Golay Correlator 32/1(In)

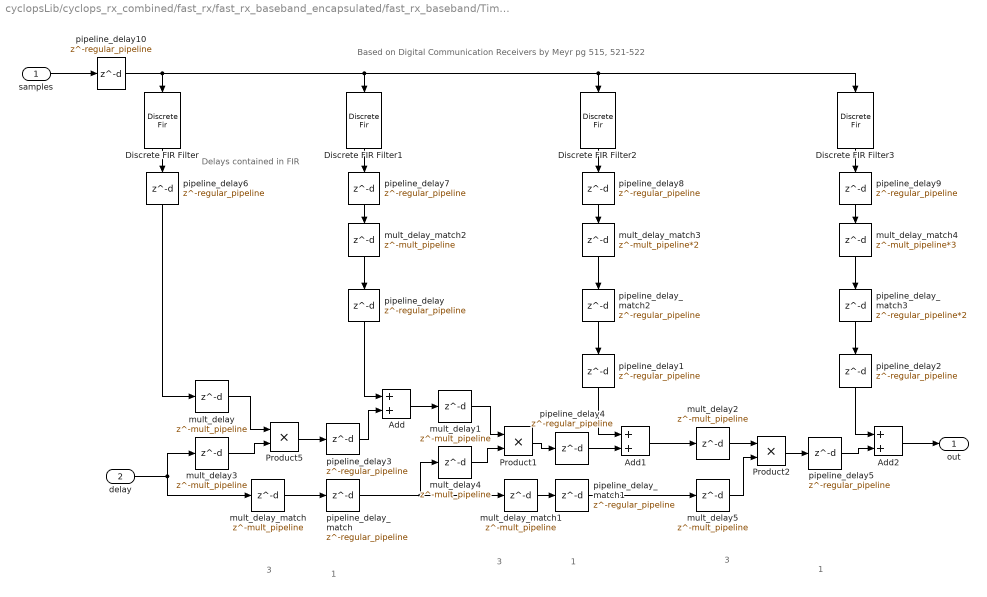
== system cyclopsLib/cyclops_rx_combined/fast_rx/fast_rx_baseband_encapsulated/fast_rx_baseband/Timing Recovery/frac_delay_farrow_N-2_M-3 ==
  note: 1
  note: 3
  note: 1
  note: 3
  note: 1
  note: 3
  note: Based on Digital Communication Receivers by Meyr pg 515, 521-522
  note: Delays contained in FIR
  samples : Inport
  delay : Inport  Port=2
  Add : Sum  OutDataTypeStr=Inherit: Same as first input
  Add1 : Sum  OutDataTypeStr=Inherit: Same as first input
  Add2 : Sum  OutDataTypeStr=Inherit: Same as first input
  Discrete FIR Filter : DiscreteFir  FilterStructure=Direct form transposed  Coefficients=[-0.22485, 0.64567, -0.64567, 0.22485]  OutDataTypeStr=Inherit: Same as input
  Discrete FIR Filter1 : DiscreteFir  FilterStructure=Direct form transposed  Coefficients=[0.70609, -1.31155, 0.62547, 0.03154]  OutDataTypeStr=Inherit: Same as input
  Discrete FIR Filter2 : DiscreteFir  FilterStructure=Direct form transposed  Coefficients=[-0.48124, -0.33413, 1.02020, -0.25639]  OutDataTypeStr=Inherit: Same as input
  Discrete FIR Filter3 : DiscreteFir  FilterStructure=Direct form transposed  Coefficients=[0, 1, 0, 0]  OutDataTypeStr=Inherit: Same as input
  Product1 : Product  OutDataTypeStr=Inherit: Same as first input
  Product2 : Product  OutDataTypeStr=Inherit: Same as first input
  Product5 : Product  OutDataTypeStr=Inherit: Same as first input
  mult_delay{,1..5} (6 alike) : Delay  DelayLength=mult_pipeline
  mult_delay_match : Delay  DelayLength=mult_pipeline
  mult_delay_match1 : Delay  DelayLength=mult_pipeline
  mult_delay_match2 : Delay  DelayLength=mult_pipeline
  mult_delay_match3 : Delay  DelayLength=mult_pipeline*2
  mult_delay_match4 : Delay  DelayLength=mult_pipeline*3
  pipeline_delay{,1..10} (11 alike) : Delay  DelayLength=regular_pipeline
  pipeline_delay_match : Delay  DelayLength=regular_pipeline
  pipeline_delay_match1 : Delay  DelayLength=regular_pipeline
  pipeline_delay_match2 : Delay  DelayLength=regular_pipeline
  pipeline_delay_match3 : Delay  DelayLength=regular_pipeline*2
  out : Outport  VectorParamsAs1DForOutWhenUnconnected=off
  wires:
  Discrete FIR Filter3/1 -> pipeline_delay9/1
  Discrete FIR Filter/1 -> pipeline_delay6/1
  delay/1 -> mult_delay3/1, mult_delay_match/1
  samples/1 -> pipeline_delay10/1
  Discrete FIR Filter1/1 -> pipeline_delay7/1
  Product5/1 -> pipeline_delay3/1
  Add/1 -> mult_delay1/1
  Discrete FIR Filter2/1 -> pipeline_delay8/1
  Add1/1 -> mult_delay2/1
  Add2/1 -> out/1
  Product1/1 -> pipeline_delay4/1
  Product2/1 -> pipeline_delay5/1
  mult_delay_match/1 -> pipeline_delay_match/1
  mult_delay_match1/1 -> pipeline_delay_match1/1
  mult_delay_match2/1 -> pipeline_delay/1
  mult_delay_match3/1 -> pipeline_delay_match2/1
  mult_delay_match4/1 -> pipeline_delay_match3/1
  mult_delay3/1 -> Product5/2
  mult_delay/1 -> Product5/1
  mult_delay1/1 -> Product1/1
  mult_delay4/1 -> Product1/2
  mult_delay2/1 -> Product2/1
  mult_delay5/1 -> Product2/2
  pipeline_delay/1 -> Add/1
  pipeline_delay3/1 -> Add/2
  pipeline_delay4/1 -> Add1/2
  pipeline_delay5/1 -> Add2/2
  pipeline_delay_match/1 -> mult_delay_match1/1, mult_delay4/1
  pipeline_delay_match1/1 -> mult_delay5/1
  pipeline_delay6/1 -> mult_delay/1
  pipeline_delay7/1 -> mult_delay_match2/1
  pipeline_delay8/1 -> mult_delay_match3/1
  pipeline_delay9/1 -> mult_delay_match4/1
  pipeline_delay10/1 -> Discrete FIR Filter/1, Discrete FIR Filter1/1, Discrete FIR Filter2/1, Discrete FIR Filter3/1
  pipeline_delay1/1 -> Add1/1
  pipeline_delay_match2/1 -> pipeline_delay1/1
  pipeline_delay2/1 -> Add2/1
  pipeline_delay_match3/1 -> pipeline_delay2/1

== system cyclopsLib/cyclops_rx_combined/fast_rx/fast_rx_baseband_encapsulated/fast_rx_baseband/Timing Recovery/sr_latch_resetNextCycle ==
  In : Inport
  set : Inport  Port=2
  rst_next : Inport  Port=3
  Constant6 : Constant  Value=0  OutDataTypeStr=single
  Delay1 : Delay  DelayLength=1
  Switch3 : Switch  Criteria=u2 > Threshold
  Switch6 : Switch  Criteria=u2 > Threshold
  Out : Outport
  wires:
  Switch3/1 -> Switch6/3, Out/1
  Delay1/1 -> Switch3/3
  Switch6/1 -> Delay1/1
  set/1 -> Switch3/2
  Constant6/1 -> Switch6/1
  In/1 -> Switch3/1
  rst_next/1 -> Switch6/2

== system cyclopsLib/cyclops_rx_combined/fast_rx/fast_rx_baseband_slim_encapsulated/slim_fast_rx/AGC/exp ==
  note: Bound Protection
  In : Inport
  Compare To Constant1 : simulink/Logic and Bit Operations/Compare To Constant  relop=>=  const=agcExpDomain  OutDataTypeStr=boolean
  Compare To Constant4 : simulink/Logic and Bit Operations/Compare To Constant  relop=<=  const=-agcExpDomain  OutDataTypeStr=boolean
  Constant11 : Constant  Value=0  OutDataTypeStr=Inherit: Inherit via back propagation  SampleTime=-1
  Constant3 : Constant  Value=exp(agcExpDomain)  OutDataTypeStr=Inherit: Inherit via back propagation  SampleTime=-1
  Constant4 : Constant  Value=exp(-agcExpDomain)  OutDataTypeStr=Inherit: Inherit via back propagation  SampleTime=-1
  Data Type Duplicate : DataTypeDuplicate
  Data Type Duplicate1 : DataTypeDuplicate
  Data Type Duplicate2 : DataTypeDuplicate
  Data Type Conversion : DataTypeConversion  OutDataTypeStr=single
  Logical Operator : Logic  Operator=OR  AllPortsSameDT=off  OutDataTypeStr=boolean
  Switch2 : Switch  Criteria=u2 ~= 0  OutDataTypeStr=Inherit: Inherit via back propagation
  Switch3 : Switch  Criteria=u2 ~= 0  OutDataTypeStr=Inherit: Inherit via back propagation
  Switch8 : Switch  Criteria=u2 ~= 0  OutDataTypeStr=Inherit: Inherit via back propagation
  exp Lookup Table : Lookup_n-D  NumberOfTableDimensions=1  BreakpointsForDimension1=[-agcExpDomain:agcExpResolution:agcExpDomain]  IndexSearchMethod=Evenly spaced points  Table=exp([-agcExpDomain:agcExpResolution:agcExpDomain])  InterpMethod=Flat  DiagnosticForOutOfRangeInput=Error  RemoveProtectionInput=on  InternalRulePriority=Speed  OutDataTypeStr=Inherit: Inherit via back propagation  RndMeth=Simplest  InputSameDT=on
  Out : Outport  VectorParamsAs1DForOutWhenUnconnected=off
  wires:
  exp Lookup Table/1 -> Data Type Duplicate2/1, Switch2/3, Data Type Duplicate/2
  Data Type Conversion/1 -> exp Lookup Table/1
  Compare To Constant4/1 -> Switch3/2, Logical Operator/2
  Compare To Constant1/1 -> Switch2/2, Logical Operator/1
  Constant11/1 -> Switch8/1
  Logical Operator/1 -> Switch8/2
  Switch3/1 -> Data Type Duplicate1/2, Data Type Duplicate2/2, Out/1
  Constant4/1 -> Switch3/1
  Switch2/1 -> Data Type Duplicate1/1, Switch3/3
  Constant3/1 -> Switch2/1
  In/1 -> Data Type Duplicate/1, Compare To Constant4/1, Compare To Constant1/1, Switch8/3
  Switch8/1 -> Data Type Conversion/1
